simulink model "doc_pnseq"  (R2014a)
settings: Solver=FixedStepDiscrete  StartTime=0.0  StopTime=125  RelTol=1e-3
libraries: commseqgen2 x3, simulink x1
settings Model: Creator=The MathWorks Inc.
settings DataIOCC: SignalLoggingSaveFormat=ModelDataLogs  SignalLoggingName=sigsOut
settings OptimizationCC: BooleanDataType=off  ExpressionDepthLimit=2147483647
settings DebuggingCC: SaveWithParameterizedLinksMsg=none  UnderspecifiedInitializationDetection=Classic  SolverPrmCheckMsg=none  MultiTaskDSMMsg=warning  MultiTaskCondExecSysMsg=none  FcnCallInpInsideContextMsg=UseLocalSettings  StateNameClashWarn=warning  StrictBusMsg=None
settings HardwareCC: ProdHWDeviceType=Specified
settings RTWCC: IncludeERTFirstTime=on
settings CodeAppCC: MangleLength=5
settings GRTTargetCC: TargetFcnLib=iso_c_tmw.mat  CombineOutputUpdateFcns=off  GRTInterface=on

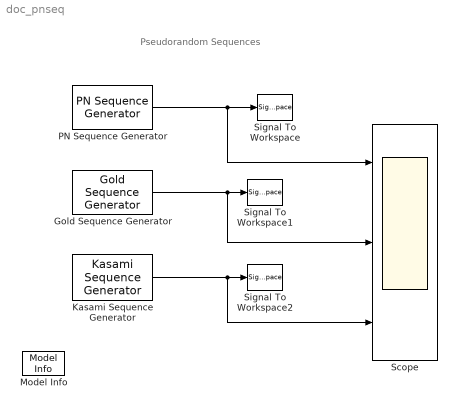
== system doc_pnseq ==
  note: Pseudorandom Sequences
  Gold Sequence Generator : commseqgen2/Gold Sequence Generator  genPoly1=[1 0 0 0 0 1 1]  iniState1=[0 0 0 0 0 1]  genPoly2=[1 1 0 0 1 1 1]  iniState2=[0 0 0 0 0 1]  index=[4]  shift=0  outVarSiz=off  maxOutSizeMode=Dialog parameter  maxOutSize=[10 1]  ts=1  frameBased=off  sampPerFrame=1  reset=off  outDataType=double
  Kasami Sequence Generator : commseqgen2/Kasami Sequence Generator  genPoly=[1 0 0 0 0 1 1]  iniState=[0 0 0 0 0 1]  codeIdx=3  shift=0  outVarSiz=off  maxOutSizeMode=Dialog parameter  maxOutSize=[10 1]  ts=1  frameBased=off  sampPerFrame=1  reset=off  outDataType=double
  Model Info : simulink/Model-Wide Utilities/Model Info  InitialBlockCM=None  BlockCM=None  Frame=on  DisplayStringWithTags=Info  HorizontalTextAlignment=Center  LeftAlignmentValue=0.5  SourceBlockDiagram=doc_pnseq  TagMaxNumber=20
  PN Sequence Generator : commseqgen2/PN Sequence Generator  poly=[1 0 0 0 0 1 1]  ini_sta=[0 0 0 0 0 1]  outBitMaskSource=Dialog parameter  shift=0  outVarSiz=off  maxOutSizeMode=Dialog parameter  maxOutSize=[10 1]  Ts=1  frameBased=off  sampPerFrame=1  reset=off  bitPackedOutputs=off  outDataType=double  numPackedBits=8  bitPackDataSigned=off  bitPackedOutDType=double
  Scope : Scope  NumInputPorts=3
      settings: YMin=-0.5~-0.5~-0.5  YMax=1.5~1.5~1.5
  Signal To Workspace : SignalToWorkspace  VariableName=pn
      settings: CopyFcn=dspblkcopystw(gcbh);  Save2DSignal=3-D array (concatenate along third dimension)
  Signal To Workspace1 : SignalToWorkspace  VariableName=gold
      settings: CopyFcn=dspblkcopystw(gcbh);  Save2DSignal=3-D array (concatenate along third dimension)
  Signal To Workspace2 : SignalToWorkspace  VariableName=kas
      settings: CopyFcn=dspblkcopystw(gcbh);  Save2DSignal=3-D array (concatenate along third dimension)
  wires:
  PN Sequence Generator/1 -> Signal To Workspace/1, Scope/1
  Gold Sequence Generator/1 -> Signal To Workspace1/1, Scope/2
  Kasami Sequence Generator/1 -> Signal To Workspace2/1, Scope/3
